simulink model "Height_Discrete_Servo_OutputFeedback"  (R2018b)
settings: Solver=VariableStepAuto  StartTime=0.0  StopTime=25  RelTol=1e-3
undefined symbols (not defined in the file): Gzd_A_obs, Gzd_B_obs, Gzd_C_obs, K0_Z, K_Z, KGe_Z, t_samp
libraries: simulink x1
settings Model: Creator=User  LastModifiedBy=User

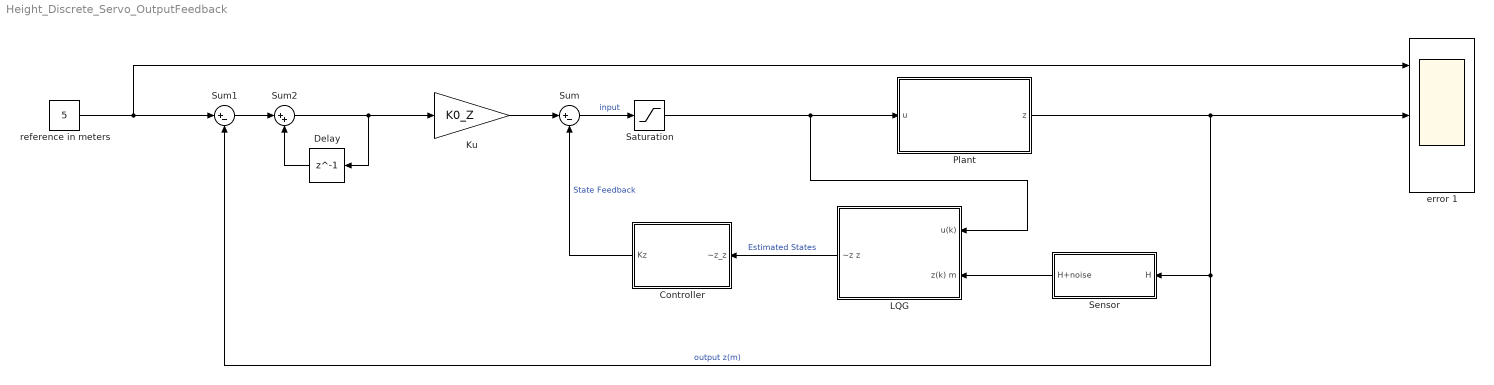
== system Height_Discrete_Servo_OutputFeedback ==
  "Controller " : Subsystem
  Delay : Delay  DelayLength=1  InitialCondition=0
  Ku : Gain  Gain=K0_Z
  LQG : Subsystem
  Plant : Subsystem
  Saturation : Saturate  UpperLimit=1.2  LowerLimit=-1.2
  Sensor : Subsystem
  Sum : Sum  Inputs=|+-
  Sum1 : Sum  Inputs=|+-
  Sum2 : Sum  Inputs=|++
  error 1 : Scope  NumInputPorts=3
  reference in meters : Constant  Value=5
  wires:
  Ku/1 -> Sum/1
  Saturation/1 -> Plant/1("u "), LQG/1(u(k))
  Sum/1 -> Saturation/1  "input"
  Plant/1("z ") -> Sum1/2, Sensor/1(H), error 1/2  "output z(m)"
  "Controller "/1(Kz) -> Sum/2  "State Feedback"
  LQG/1("~z z ") -> "Controller "/1(~z_z)  "Estimated States"
  Sensor/1(H+noise) -> LQG/2(z(k) m)
  Sum1/1 -> Sum2/1
  Delay/1 -> Sum2/2
  reference in meters/1 -> error 1/1, Sum1/1
  Sum2/1 -> Ku/1, Delay/1

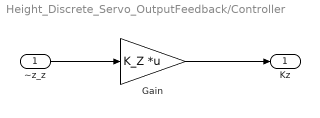
== system Height_Discrete_Servo_OutputFeedback/Controller  ==
  ~z_z : Inport
  Gain : Gain  Gain=K_Z  Multiplication=Matrix(K*u) (u vector)
  Kz : Outport
  wires:
  ~z_z/1 -> Gain/1
  Gain/1 -> Kz/1

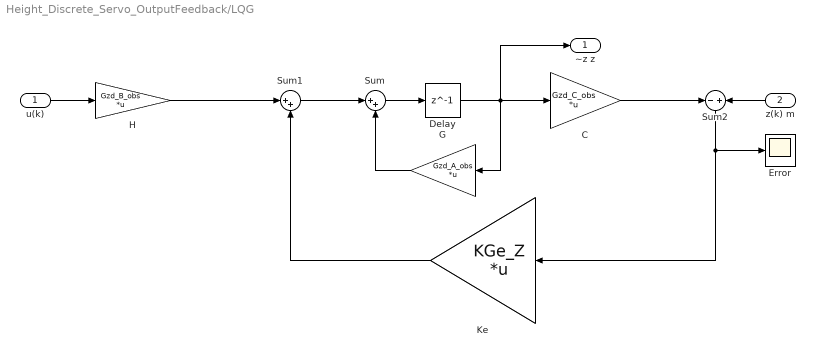
== system Height_Discrete_Servo_OutputFeedback/LQG ==
  u(k) : Inport
  z(k) m : Inport  Port=2
  C : Gain  Gain=Gzd_C_obs  Multiplication=Matrix(K*u)
  Delay : Delay  DelayLength=1  InitialCondition=0  SampleTime=t_samp
  Error : Scope
  G : Gain  Gain=Gzd_A_obs  Multiplication=Matrix(K*u)
  H : Gain  Gain=Gzd_B_obs  Multiplication=Matrix(K*u)
  Ke : Gain  Gain=KGe_Z  Multiplication=Matrix(K*u)
  Sum : Sum  Inputs=|++
  Sum1 : Sum  Inputs=|++
  Sum2 : Sum  Inputs=-+
  "~z z " : Outport
  wires:
  C/1 -> Sum2/1
  z(k) m/1 -> Sum2/2
  H/1 -> Sum1/1
  Sum/1 -> Delay/1
  u(k)/1 -> H/1
  G/1 -> Sum/2
  Sum2/1 -> Ke/1, Error/1
  Sum1/1 -> Sum/1
  Ke/1 -> Sum1/2
  Delay/1 -> G/1, "~z z "/1, C/1

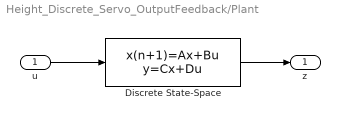
== system Height_Discrete_Servo_OutputFeedback/Plant ==
  "u " : Inport
  Discrete State-Space : DiscreteStateSpace  A=Gzd_A_obs  B=Gzd_B_obs  C=Gzd_C_obs  D=0  SampleTime=t_samp
  "z " : Outport
  wires:
  "u "/1 -> Discrete State-Space/1
  Discrete State-Space/1 -> "z "/1

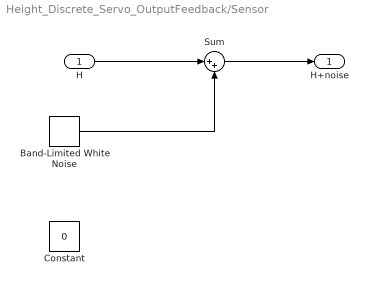
== system Height_Discrete_Servo_OutputFeedback/Sensor ==
  H : Inport
  Band-Limited White Noise : simulink/Sources/Band-Limited White Noise  Cov=.000001  Ts=0.1  seed=[124123]
  Constant : Constant  Value=0
  Sum : Sum  Inputs=|++
  H+noise : Outport
  wires:
  Sum/1 -> H+noise/1
  H/1 -> Sum/1
  Band-Limited White Noise/1 -> Sum/2
